simulink model "LUT_liver_pancreas_30"  (R2023b)
settings: Solver=FixedStepAuto  StartTime=0  StopTime=10.1  FixedStep=Timegap  RelTol=1e-3
model workspace (MAT data in the model file):
  T1_input = 1.34
(part 1 of 3)
settings Model: Creator=ppxmr2  LastModifiedBy=ppxmr2

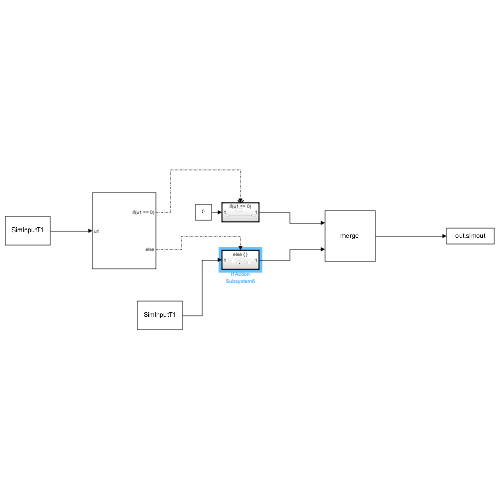
[thumbnail: Simulink's stored preview of the top-level diagram]
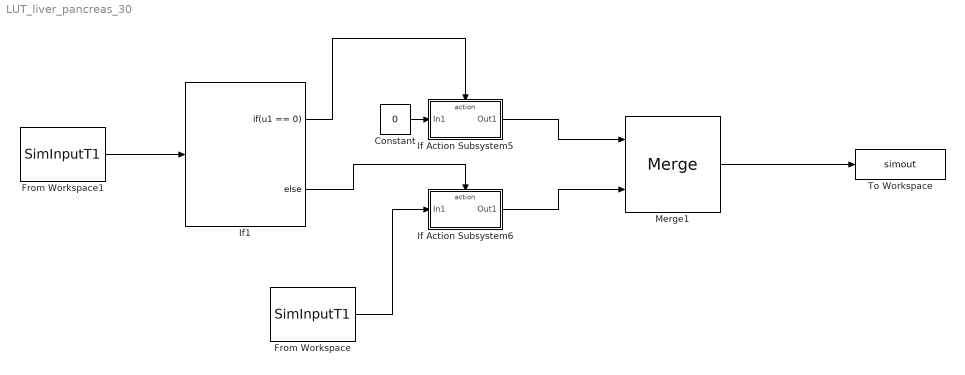
== system LUT_liver_pancreas_30 ==
  Constant : Constant  Value=0
  From Workspace : FromWorkspace  VariableName=SimInputT1  Interpolate=off  OutputAfterFinalValue=Setting to zero
  From Workspace1 : FromWorkspace  VariableName=SimInputT1  Interpolate=off  OutputAfterFinalValue=Setting to zero
  If Action Subsystem5 : Subsystem  TreatAsAtomicUnit=on
  If Action Subsystem6 : Subsystem  TreatAsAtomicUnit=on
  If1 : If  IfExpression=u1 == 0
  Merge1 : Merge
  To Workspace : ToWorkspace  VariableName=simout
  wires:
  From Workspace1/1 -> If1/1
  If1/1 -> If Action Subsystem5/Action
  If1/2 -> If Action Subsystem6/Action
  Constant/1 -> If Action Subsystem5/1(In1)
  If Action Subsystem5/1(Out1) -> Merge1/1
  If Action Subsystem6/1(Out1) -> Merge1/2
  Merge1/1 -> To Workspace/1
  From Workspace/1 -> If Action Subsystem6/1(In1)

== system LUT_liver_pancreas_30/If Action Subsystem5 ==
  In1 : Inport
  Action Port : ActionPort  ActionPortLabel=if(u1 == 0)
  Out1 : Outport
  wires:
  In1/1 -> Out1/1

== system LUT_liver_pancreas_30/If Action Subsystem6 ==
  In1 : Inport
  Action Port : ActionPort  ActionPortLabel=else
  From Workspace1 : FromWorkspace  VariableName=SimInputHR  Interpolate=off  OutputAfterFinalValue=Setting to zero
  If : If  IfExpression=u1 >= 1.495  ElseIfExpressions=u1 >= 0.995
  If Action Subsystem1 : Subsystem  TreatAsAtomicUnit=on
  If Action Subsystem2 : Subsystem  TreatAsAtomicUnit=on
  If Action Subsystem3 : Subsystem  TreatAsAtomicUnit=on
  Merge : Merge  Inputs=3
  Out1 : Outport
  wires:
  Merge/1 -> Out1/1
  From Workspace1/1 -> If/1
  If Action Subsystem1/1(Out1) -> Merge/2
  If Action Subsystem3/1(Out1) -> Merge/3
  In1/1 -> If Action Subsystem2/1(In1), If Action Subsystem1/1(In1), If Action Subsystem3/1(In1)
  If/1 -> If Action Subsystem2/Action
  If/2 -> If Action Subsystem1/Action
  If/3 -> If Action Subsystem3/Action
  If Action Subsystem2/1(Out1) -> Merge/1

== system LUT_liver_pancreas_30/If Action Subsystem6/If Action Subsystem1 ==
  In1 : Inport
  Action Port : ActionPort  ActionPortLabel=elseif(u1 >= 0.995)
  From Workspace2 : FromWorkspace  VariableName=SimInputHR  Interpolate=off  OutputAfterFinalValue=Setting to zero
  If Action Subsystem5 : Subsystem  TreatAsAtomicUnit=on
  If Action Subsystem6 : Subsystem  TreatAsAtomicUnit=on
  If Action Subsystem7 : Subsystem  TreatAsAtomicUnit=on
  If Action Subsystem8 : Subsystem  TreatAsAtomicUnit=on
  If Action Subsystem9 : Subsystem  TreatAsAtomicUnit=on
  If1 : If  IfExpression=u1 >= 1.395  ElseIfExpressions=u1 >= 1.295, u1 >= 1.195, u1 >= 1.095
  Merge1 : Merge  Inputs=5
  Out1 : Outport
  wires:
  In1/1 -> If Action Subsystem7/1(In2), If Action Subsystem8/1(In1), If Action Subsystem9/1(In1), If Action Subsystem5/1(In1), If Action Subsystem6/1(In1)
  From Workspace2/1 -> If1/1
  If Action Subsystem9/1(Out1) -> Merge1/1
  If Action Subsystem6/1(Out1) -> Merge1/5
  If Action Subsystem8/1(Out1) -> Merge1/2
  If Action Subsystem5/1(Out1) -> Merge1/4
  If1/4 -> If Action Subsystem5/Action
  If1/2 -> If Action Subsystem8/Action
  If1/3 -> If Action Subsystem7/Action
  If Action Subsystem7/1(Out2) -> Merge1/3
  If1/5 -> If Action Subsystem6/Action
  If1/1 -> If Action Subsystem9/Action
  Merge1/1 -> Out1/1

== system LUT_liver_pancreas_30/If Action Subsystem6/If Action Subsystem2 ==
  In1 : Inport
  Action Port : ActionPort  ActionPortLabel=if(u1 >= 1.495)
  From Workspace2 : FromWorkspace  VariableName=SimInputHR  Interpolate=off  OutputAfterFinalValue=Setting to zero
  If Action Subsystem5 : Subsystem  TreatAsAtomicUnit=on
  If Action Subsystem6 : Subsystem  TreatAsAtomicUnit=on
  If Action Subsystem7 : Subsystem  TreatAsAtomicUnit=on
  If Action Subsystem8 : Subsystem  TreatAsAtomicUnit=on
  If Action Subsystem9 : Subsystem  TreatAsAtomicUnit=on
  If1 : If  IfExpression=u1 >= 1.895  ElseIfExpressions=u1 >= 1.795, u1 >= 1.695, u1 >= 1.595
  Merge1 : Merge  Inputs=5
  Out1 : Outport
  wires:
  In1/1 -> If Action Subsystem9/1(In1), If Action Subsystem8/1(In1), If Action Subsystem7/1(In1), If Action Subsystem5/1(In1), If Action Subsystem6/1(In1)
  From Workspace2/1 -> If1/1
  If Action Subsystem9/1(Out1) -> Merge1/1
  If1/4 -> If Action Subsystem5/Action
  If1/2 -> If Action Subsystem8/Action
  If1/3 -> If Action Subsystem7/Action
  If1/5 -> If Action Subsystem6/Action
  If1/1 -> If Action Subsystem9/Action
  Merge1/1 -> Out1/1
  If Action Subsystem8/1(Out1) -> Merge1/2
  If Action Subsystem7/1(Out1) -> Merge1/3
  If Action Subsystem6/1(Out1) -> Merge1/5
  If Action Subsystem5/1(Out1) -> Merge1/4

== system LUT_liver_pancreas_30/If Action Subsystem6/If Action Subsystem3 ==
  In1 : Inport
  Action Port : ActionPort  ActionPortLabel=else
  From Workspace2 : FromWorkspace  VariableName=SimInputHR  Interpolate=off  OutputAfterFinalValue=Setting to zero
  If Action Subsystem5 : Subsystem  TreatAsAtomicUnit=on
  If Action Subsystem6 : Subsystem  TreatAsAtomicUnit=on
  If Action Subsystem7 : Subsystem  TreatAsAtomicUnit=on
  If Action Subsystem8 : Subsystem  TreatAsAtomicUnit=on
  If Action Subsystem9 : Subsystem  TreatAsAtomicUnit=on
  If1 : If  IfExpression=u1 >= 0.895  ElseIfExpressions=u1 >= 0.795, u1 >= 0.695, u1 >= 0595
  Merge1 : Merge  Inputs=5
  Out1 : Outport
  wires:
  In1/1 -> If Action Subsystem8/1(In1), If Action Subsystem9/1(In2), If Action Subsystem7/1(In1), If Action Subsystem5/1(In1), If Action Subsystem6/1(In1)
  From Workspace2/1 -> If1/1
  If Action Subsystem9/1(Out2) -> Merge1/1
  If Action Subsystem6/1(Out1) -> Merge1/5
  If Action Subsystem8/1(Out1) -> Merge1/2
  If Action Subsystem5/1(Out1) -> Merge1/4
  If1/4 -> If Action Subsystem5/Action
  If1/2 -> If Action Subsystem8/Action
  If1/3 -> If Action Subsystem7/Action
  If Action Subsystem7/1(Out1) -> Merge1/3
  If1/5 -> If Action Subsystem6/Action
  If1/1 -> If Action Subsystem9/Action
  Merge1/1 -> Out1/1

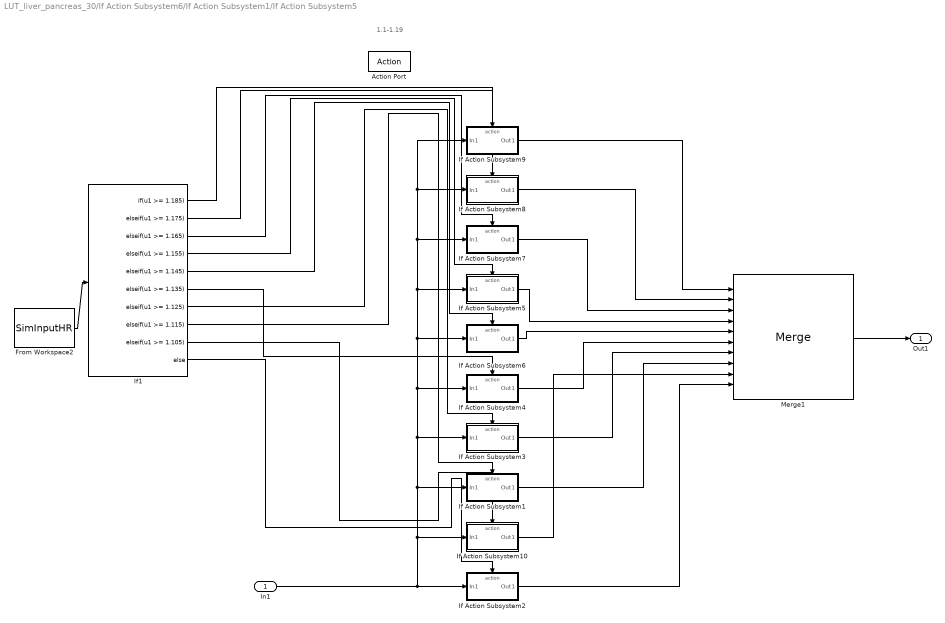
== system LUT_liver_pancreas_30/If Action Subsystem6/If Action Subsystem1/If Action Subsystem5 ==
  note: 1.1-1.19
  In1 : Inport
  Action Port : ActionPort  ActionPortLabel=elseif( u1 >= 1.095)
  From Workspace2 : FromWorkspace  VariableName=SimInputHR  Interpolate=off  OutputAfterFinalValue=Setting to zero
  If Action Subsystem1 : Subsystem  TreatAsAtomicUnit=on
  If Action Subsystem10 : Subsystem  TreatAsAtomicUnit=on
  If Action Subsystem2 : Subsystem  TreatAsAtomicUnit=on
  If Action Subsystem3 : Subsystem  TreatAsAtomicUnit=on
  If Action Subsystem4 : Subsystem  TreatAsAtomicUnit=on
  If Action Subsystem5 : Subsystem  TreatAsAtomicUnit=on
  If Action Subsystem6 : Subsystem  TreatAsAtomicUnit=on
  If Action Subsystem7 : Subsystem  TreatAsAtomicUnit=on
  If Action Subsystem8 : Subsystem  TreatAsAtomicUnit=on
  If Action Subsystem9 : Subsystem  TreatAsAtomicUnit=on
  If1 : If  IfExpression=u1 >= 1.185  ElseIfExpressions=u1 >= 1.175, u1 >= 1.165, u1 >= 1.155, u1 >= 1.145, u1 >= 1.135, u1 >= 1.125, u1 >= 1.115, u1 >= 1.105
  Merge1 : Merge  Inputs=10
  Out1 : Outport
  wires:
  If1/10 -> If Action Subsystem2/Action
  If Action Subsystem4/1(Out1) -> Merge1/6
  From Workspace2/1 -> If1/1
  If Action Subsystem6/1(Out1) -> Merge1/5
  Merge1/1 -> Out1/1
  If1/8 -> If Action Subsystem1/Action
  If Action Subsystem3/1(Out1) -> Merge1/7
  In1/1 -> If Action Subsystem1/1(In1), If Action Subsystem3/1(In1), If Action Subsystem7/1(In1), If Action Subsystem8/1(In1), If Action Subsystem9/1(In1), If Action Subsystem5/1(In1), If Action Subsystem6/1(In1), If Action Subsystem4/1(In1), If Action Subsystem10/1(In1), If Action Subsystem2/1(In1)
  If1/6 -> If Action Subsystem4/Action
  If Action Subsystem1/1(Out1) -> Merge1/8
  If1/4 -> If Action Subsystem5/Action
  If Action Subsystem8/1(Out1) -> Merge1/2
  If1/5 -> If Action Subsystem6/Action
  If Action Subsystem7/1(Out1) -> Merge1/3
  If1/3 -> If Action Subsystem7/Action
  If1/7 -> If Action Subsystem3/Action
  If Action Subsystem5/1(Out1) -> Merge1/4
  If Action Subsystem2/1(Out1) -> Merge1/10
  If1/2 -> If Action Subsystem8/Action
  If1/1 -> If Action Subsystem9/Action
  If Action Subsystem9/1(Out1) -> Merge1/1
  If1/9 -> If Action Subsystem10/Action
  If Action Subsystem10/1(Out1) -> Merge1/9

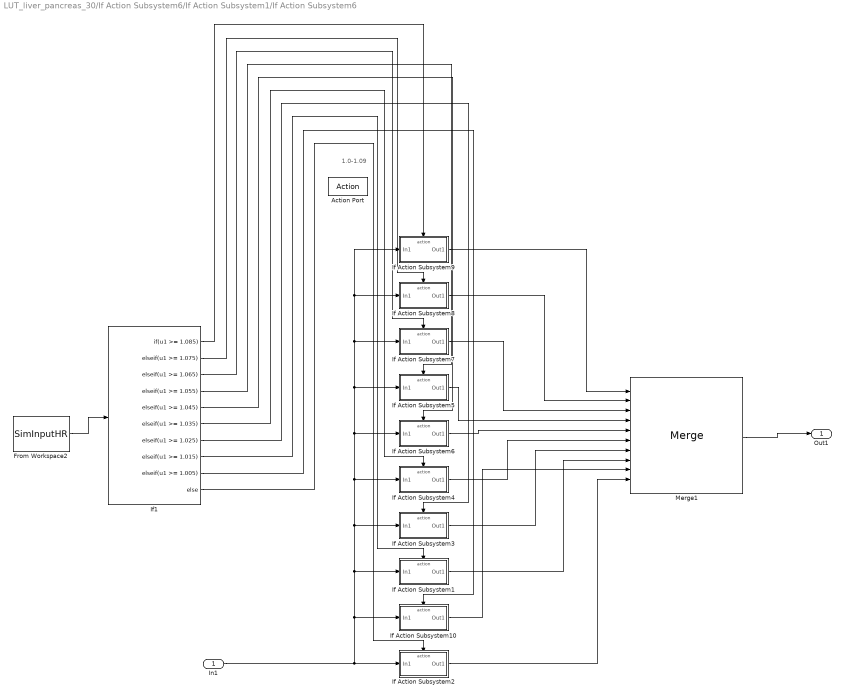
== system LUT_liver_pancreas_30/If Action Subsystem6/If Action Subsystem1/If Action Subsystem6 ==
  note: 1.0-1.09
  In1 : Inport
  Action Port : ActionPort  ActionPortLabel=else
  From Workspace2 : FromWorkspace  VariableName=SimInputHR  Interpolate=off  OutputAfterFinalValue=Setting to zero
  If Action Subsystem1 : Subsystem  TreatAsAtomicUnit=on
  If Action Subsystem10 : Subsystem  TreatAsAtomicUnit=on
  If Action Subsystem2 : Subsystem  TreatAsAtomicUnit=on
  If Action Subsystem3 : Subsystem  TreatAsAtomicUnit=on
  If Action Subsystem4 : Subsystem  TreatAsAtomicUnit=on
  If Action Subsystem5 : Subsystem  TreatAsAtomicUnit=on
  If Action Subsystem6 : Subsystem  TreatAsAtomicUnit=on
  If Action Subsystem7 : Subsystem  TreatAsAtomicUnit=on
  If Action Subsystem8 : Subsystem  TreatAsAtomicUnit=on
  If Action Subsystem9 : Subsystem  TreatAsAtomicUnit=on
  If1 : If  IfExpression=u1 >= 1.085  ElseIfExpressions=u1 >= 1.075, u1 >= 1.065, u1 >= 1.055, u1 >= 1.045, u1 >= 1.035, u1 >= 1.025, u1 >= 1.015, u1 >= 1.005
  Merge1 : Merge  Inputs=10
  Out1 : Outport
  wires:
  If1/10 -> If Action Subsystem2/Action
  If Action Subsystem4/1(Out1) -> Merge1/6
  From Workspace2/1 -> If1/1
  If Action Subsystem6/1(Out1) -> Merge1/5
  Merge1/1 -> Out1/1
  If1/8 -> If Action Subsystem1/Action
  If Action Subsystem3/1(Out1) -> Merge1/7
  In1/1 -> If Action Subsystem1/1(In1), If Action Subsystem3/1(In1), If Action Subsystem4/1(In1), If Action Subsystem7/1(In1), If Action Subsystem8/1(In1), If Action Subsystem9/1(In1), If Action Subsystem5/1(In1), If Action Subsystem6/1(In1), If Action Subsystem10/1(In1), If Action Subsystem2/1(In1)
  If1/6 -> If Action Subsystem4/Action
  If Action Subsystem1/1(Out1) -> Merge1/8
  If1/4 -> If Action Subsystem5/Action
  If Action Subsystem8/1(Out1) -> Merge1/2
  If1/5 -> If Action Subsystem6/Action
  If Action Subsystem7/1(Out1) -> Merge1/3
  If1/3 -> If Action Subsystem7/Action
  If1/7 -> If Action Subsystem3/Action
  If Action Subsystem5/1(Out1) -> Merge1/4
  If Action Subsystem2/1(Out1) -> Merge1/10
  If1/2 -> If Action Subsystem8/Action
  If1/1 -> If Action Subsystem9/Action
  If Action Subsystem9/1(Out1) -> Merge1/1
  If1/9 -> If Action Subsystem10/Action
  If Action Subsystem10/1(Out1) -> Merge1/9

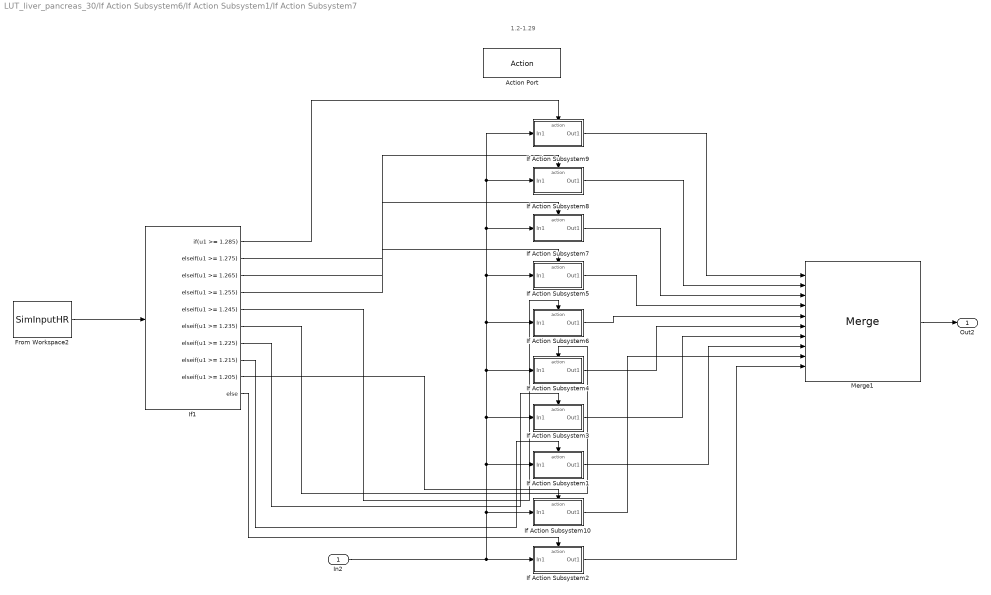
== system LUT_liver_pancreas_30/If Action Subsystem6/If Action Subsystem1/If Action Subsystem7 ==
  note: 1.2-1.29
  In2 : Inport
  Action Port : ActionPort  ActionPortLabel=elseif( u1 >= 1.195)
  From Workspace2 : FromWorkspace  VariableName=SimInputHR  Interpolate=off  OutputAfterFinalValue=Setting to zero
  If Action Subsystem1 : Subsystem  TreatAsAtomicUnit=on
  If Action Subsystem10 : Subsystem  TreatAsAtomicUnit=on
  If Action Subsystem2 : Subsystem  TreatAsAtomicUnit=on
  If Action Subsystem3 : Subsystem  TreatAsAtomicUnit=on
  If Action Subsystem4 : Subsystem  TreatAsAtomicUnit=on
  If Action Subsystem5 : Subsystem  TreatAsAtomicUnit=on
  If Action Subsystem6 : Subsystem  TreatAsAtomicUnit=on
  If Action Subsystem7 : Subsystem  TreatAsAtomicUnit=on
  If Action Subsystem8 : Subsystem  TreatAsAtomicUnit=on
  If Action Subsystem9 : Subsystem  TreatAsAtomicUnit=on
  If1 : If  IfExpression=u1 >= 1.285  ElseIfExpressions=u1 >= 1.275, u1 >= 1.265, u1 >= 1.255, u1 >= 1.245, u1 >= 1.235, u1 >= 1.225, u1 >= 1.215, u1 >= 1.205
  Merge1 : Merge  Inputs=10
  Out2 : Outport
  wires:
  If1/10 -> If Action Subsystem2/Action
  If Action Subsystem4/1(Out1) -> Merge1/6
  From Workspace2/1 -> If1/1
  If Action Subsystem6/1(Out1) -> Merge1/5
  Merge1/1 -> Out2/1
  If1/8 -> If Action Subsystem1/Action
  If Action Subsystem3/1(Out1) -> Merge1/7
  In2/1 -> If Action Subsystem1/1(In1), If Action Subsystem3/1(In1), If Action Subsystem4/1(In1), If Action Subsystem7/1(In1), If Action Subsystem8/1(In1), If Action Subsystem9/1(In1), If Action Subsystem5/1(In1), If Action Subsystem6/1(In1), If Action Subsystem10/1(In1), If Action Subsystem2/1(In1)
  If1/6 -> If Action Subsystem4/Action
  If Action Subsystem1/1(Out1) -> Merge1/8
  If1/4 -> If Action Subsystem5/Action
  If Action Subsystem8/1(Out1) -> Merge1/2
  If1/5 -> If Action Subsystem6/Action
  If Action Subsystem7/1(Out1) -> Merge1/3
  If1/3 -> If Action Subsystem7/Action
  If1/7 -> If Action Subsystem3/Action
  If Action Subsystem5/1(Out1) -> Merge1/4
  If Action Subsystem2/1(Out1) -> Merge1/10
  If1/2 -> If Action Subsystem8/Action
  If1/1 -> If Action Subsystem9/Action
  If Action Subsystem9/1(Out1) -> Merge1/1
  If Action Subsystem10/1(Out1) -> Merge1/9
  If1/9 -> If Action Subsystem10/Action

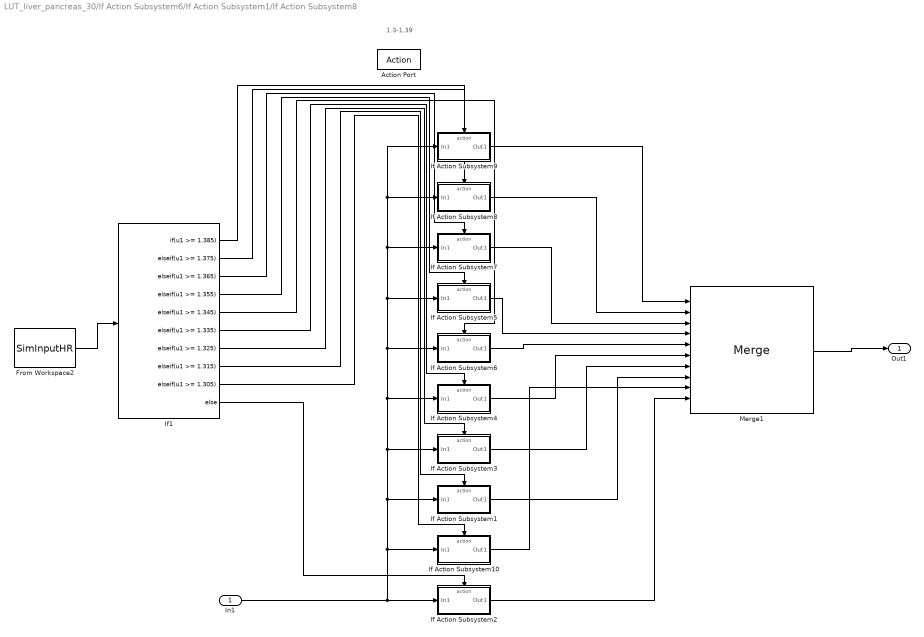
== system LUT_liver_pancreas_30/If Action Subsystem6/If Action Subsystem1/If Action Subsystem8 ==
  note: 1.3-1.39
  In1 : Inport
  Action Port : ActionPort  ActionPortLabel=elseif(u1 >= 1.295)
  From Workspace2 : FromWorkspace  VariableName=SimInputHR  Interpolate=off  OutputAfterFinalValue=Setting to zero
  If Action Subsystem1 : Subsystem  TreatAsAtomicUnit=on
  If Action Subsystem10 : Subsystem  TreatAsAtomicUnit=on
  If Action Subsystem2 : Subsystem  TreatAsAtomicUnit=on
  If Action Subsystem3 : Subsystem  TreatAsAtomicUnit=on
  If Action Subsystem4 : Subsystem  TreatAsAtomicUnit=on
  If Action Subsystem5 : Subsystem  TreatAsAtomicUnit=on
  If Action Subsystem6 : Subsystem  TreatAsAtomicUnit=on
  If Action Subsystem7 : Subsystem  TreatAsAtomicUnit=on
  If Action Subsystem8 : Subsystem  TreatAsAtomicUnit=on
  If Action Subsystem9 : Subsystem  TreatAsAtomicUnit=on
  If1 : If  IfExpression=u1 >= 1.385  ElseIfExpressions=u1 >= 1.375, u1 >= 1.365, u1 >= 1.355, u1 >= 1.345, u1 >= 1.335, u1 >= 1.325, u1 >= 1.315, u1 >= 1.305
  Merge1 : Merge  Inputs=10
  Out1 : Outport
  wires:
  If1/10 -> If Action Subsystem2/Action
  If Action Subsystem4/1(Out1) -> Merge1/6
  From Workspace2/1 -> If1/1
  If Action Subsystem6/1(Out1) -> Merge1/5
  Merge1/1 -> Out1/1
  If1/8 -> If Action Subsystem1/Action
  If Action Subsystem3/1(Out1) -> Merge1/7
  In1/1 -> If Action Subsystem1/1(In1), If Action Subsystem3/1(In1), If Action Subsystem4/1(In1), If Action Subsystem7/1(In1), If Action Subsystem8/1(In1), If Action Subsystem9/1(In1), If Action Subsystem5/1(In1), If Action Subsystem6/1(In1), If Action Subsystem10/1(In1), If Action Subsystem2/1(In1)
  If1/6 -> If Action Subsystem4/Action
  If Action Subsystem1/1(Out1) -> Merge1/8
  If1/4 -> If Action Subsystem5/Action
  If Action Subsystem8/1(Out1) -> Merge1/2
  If1/5 -> If Action Subsystem6/Action
  If Action Subsystem7/1(Out1) -> Merge1/3
  If1/3 -> If Action Subsystem7/Action
  If1/7 -> If Action Subsystem3/Action
  If Action Subsystem5/1(Out1) -> Merge1/4
  If Action Subsystem2/1(Out1) -> Merge1/10
  If1/2 -> If Action Subsystem8/Action
  If1/1 -> If Action Subsystem9/Action
  If Action Subsystem9/1(Out1) -> Merge1/1
  If1/9 -> If Action Subsystem10/Action
  If Action Subsystem10/1(Out1) -> Merge1/9

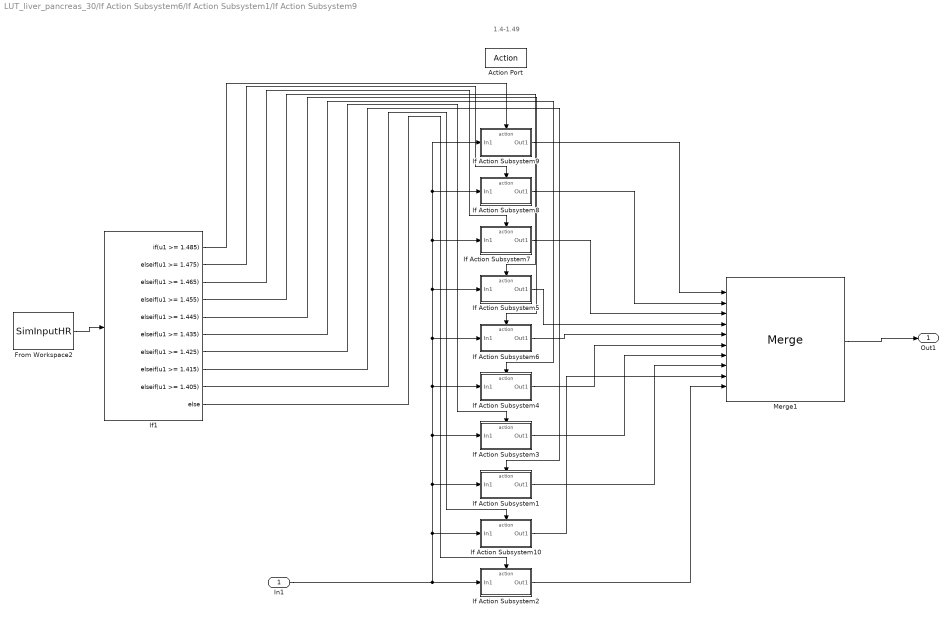
== system LUT_liver_pancreas_30/If Action Subsystem6/If Action Subsystem1/If Action Subsystem9 ==
  note: 1.4-1.49
  In1 : Inport
  Action Port : ActionPort  ActionPortLabel=if(u1 >= 1.395)
  From Workspace2 : FromWorkspace  VariableName=SimInputHR  Interpolate=off  OutputAfterFinalValue=Setting to zero
  If Action Subsystem1 : Subsystem  TreatAsAtomicUnit=on
  If Action Subsystem10 : Subsystem  TreatAsAtomicUnit=on
  If Action Subsystem2 : Subsystem  TreatAsAtomicUnit=on
  If Action Subsystem3 : Subsystem  TreatAsAtomicUnit=on
  If Action Subsystem4 : Subsystem  TreatAsAtomicUnit=on
  If Action Subsystem5 : Subsystem  TreatAsAtomicUnit=on
  If Action Subsystem6 : Subsystem  TreatAsAtomicUnit=on
  If Action Subsystem7 : Subsystem  TreatAsAtomicUnit=on
  If Action Subsystem8 : Subsystem  TreatAsAtomicUnit=on
  If Action Subsystem9 : Subsystem  TreatAsAtomicUnit=on
  If1 : If  IfExpression=u1 >= 1.485  ElseIfExpressions=u1 >= 1.475, u1 >= 1.465, u1 >= 1.455, u1 >= 1.445, u1 >= 1.435, u1 >= 1.425, u1 >= 1.415, u1 >= 1.405
  Merge1 : Merge  Inputs=10
  Out1 : Outport
  wires:
  If1/10 -> If Action Subsystem2/Action
  If Action Subsystem4/1(Out1) -> Merge1/6
  From Workspace2/1 -> If1/1
  If Action Subsystem6/1(Out1) -> Merge1/5
  Merge1/1 -> Out1/1
  If1/8 -> If Action Subsystem1/Action
  If Action Subsystem3/1(Out1) -> Merge1/7
  In1/1 -> If Action Subsystem10/1(In1), If Action Subsystem1/1(In1), If Action Subsystem3/1(In1), If Action Subsystem4/1(In1), If Action Subsystem7/1(In1), If Action Subsystem8/1(In1), If Action Subsystem9/1(In1), If Action Subsystem5/1(In1), If Action Subsystem6/1(In1), If Action Subsystem2/1(In1)
  If1/6 -> If Action Subsystem4/Action
  If Action Subsystem1/1(Out1) -> Merge1/8
  If1/4 -> If Action Subsystem5/Action
  If Action Subsystem8/1(Out1) -> Merge1/2
  If1/5 -> If Action Subsystem6/Action
  If Action Subsystem7/1(Out1) -> Merge1/3
  If1/3 -> If Action Subsystem7/Action
  If1/7 -> If Action Subsystem3/Action
  If Action Subsystem5/1(Out1) -> Merge1/4
  If Action Subsystem2/1(Out1) -> Merge1/10
  If1/2 -> If Action Subsystem8/Action
  If1/1 -> If Action Subsystem9/Action
  If Action Subsystem9/1(Out1) -> Merge1/1
  If1/9 -> If Action Subsystem10/Action
  If Action Subsystem10/1(Out1) -> Merge1/9

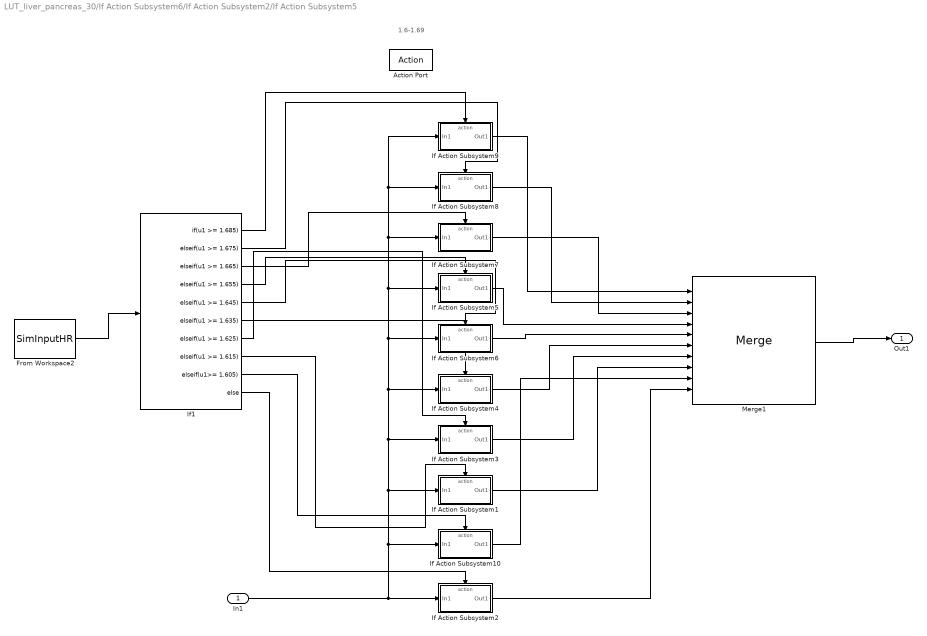
== system LUT_liver_pancreas_30/If Action Subsystem6/If Action Subsystem2/If Action Subsystem5 ==
  note: 1.6-1.69
  In1 : Inport
  Action Port : ActionPort  ActionPortLabel=elseif( u1 >= 1.595)
  From Workspace2 : FromWorkspace  VariableName=SimInputHR  Interpolate=off  OutputAfterFinalValue=Setting to zero
  If Action Subsystem1 : Subsystem  TreatAsAtomicUnit=on
  If Action Subsystem10 : Subsystem  TreatAsAtomicUnit=on
  If Action Subsystem2 : Subsystem  TreatAsAtomicUnit=on
  If Action Subsystem3 : Subsystem  TreatAsAtomicUnit=on
  If Action Subsystem4 : Subsystem  TreatAsAtomicUnit=on
  If Action Subsystem5 : Subsystem  TreatAsAtomicUnit=on
  If Action Subsystem6 : Subsystem  TreatAsAtomicUnit=on
  If Action Subsystem7 : Subsystem  TreatAsAtomicUnit=on
  If Action Subsystem8 : Subsystem  TreatAsAtomicUnit=on
  If Action Subsystem9 : Subsystem  TreatAsAtomicUnit=on
  If1 : If  IfExpression=u1 >= 1.685  ElseIfExpressions=u1 >= 1.675, u1 >= 1.665, u1 >= 1.655, u1 >= 1.645, u1 >= 1.635, u1 >= 1.625, u1 >= 1.615, u1>= 1.605
  Merge1 : Merge  Inputs=10
  Out1 : Outport
  wires:
  If1/2 -> If Action Subsystem8/Action
  If Action Subsystem5/1(Out1) -> Merge1/4
  If1/3 -> If Action Subsystem7/Action
  If Action Subsystem9/1(Out1) -> Merge1/1
  If1/7 -> If Action Subsystem3/Action
  If1/5 -> If Action Subsystem6/Action
  If1/1 -> If Action Subsystem9/Action
  If Action Subsystem4/1(Out1) -> Merge1/6
  If1/10 -> If Action Subsystem2/Action
  If Action Subsystem8/1(Out1) -> Merge1/2
  If1/4 -> If Action Subsystem5/Action
  In1/1 -> If Action Subsystem10/1(In1), If Action Subsystem1/1(In1), If Action Subsystem3/1(In1), If Action Subsystem4/1(In1), If Action Subsystem7/1(In1), If Action Subsystem8/1(In1), If Action Subsystem9/1(In1), If Action Subsystem5/1(In1), If Action Subsystem6/1(In1), If Action Subsystem2/1(In1)
  If Action Subsystem1/1(Out1) -> Merge1/8
  If Action Subsystem2/1(Out1) -> Merge1/10
  If1/8 -> If Action Subsystem1/Action
  If Action Subsystem3/1(Out1) -> Merge1/7
  If1/6 -> If Action Subsystem4/Action
  From Workspace2/1 -> If1/1
  Merge1/1 -> Out1/1
  If Action Subsystem6/1(Out1) -> Merge1/5
  If Action Subsystem7/1(Out1) -> Merge1/3
  If1/9 -> If Action Subsystem10/Action
  If Action Subsystem10/1(Out1) -> Merge1/9

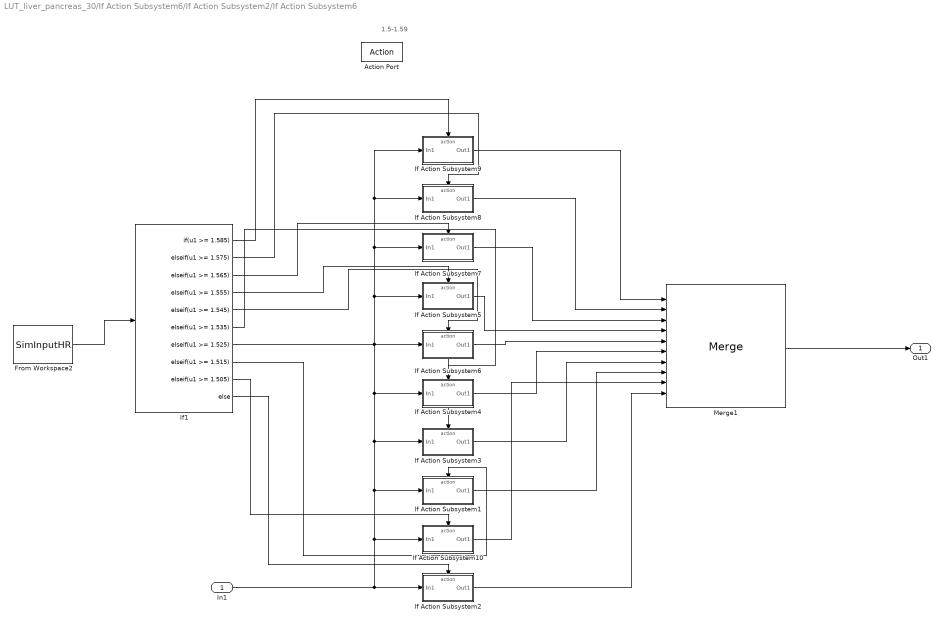
== system LUT_liver_pancreas_30/If Action Subsystem6/If Action Subsystem2/If Action Subsystem6 ==
  note: 1.5-1.59
  In1 : Inport
  Action Port : ActionPort  ActionPortLabel=else
  From Workspace2 : FromWorkspace  VariableName=SimInputHR  Interpolate=off  OutputAfterFinalValue=Setting to zero
  If Action Subsystem1 : Subsystem  TreatAsAtomicUnit=on
  If Action Subsystem10 : Subsystem  TreatAsAtomicUnit=on
  If Action Subsystem2 : Subsystem  TreatAsAtomicUnit=on
  If Action Subsystem3 : Subsystem  TreatAsAtomicUnit=on
  If Action Subsystem4 : Subsystem  TreatAsAtomicUnit=on
  If Action Subsystem5 : Subsystem  TreatAsAtomicUnit=on
  If Action Subsystem6 : Subsystem  TreatAsAtomicUnit=on
  If Action Subsystem7 : Subsystem  TreatAsAtomicUnit=on
  If Action Subsystem8 : Subsystem  TreatAsAtomicUnit=on
  If Action Subsystem9 : Subsystem  TreatAsAtomicUnit=on
  If1 : If  IfExpression=u1 >= 1.585  ElseIfExpressions=u1 >= 1.575, u1 >= 1.565, u1 >= 1.555, u1 >= 1.545, u1 >= 1.535, u1 >= 1.525, u1 >= 1.515, u1 >= 1.505
  Merge1 : Merge  Inputs=10
  Out1 : Outport
  wires:
  If1/2 -> If Action Subsystem8/Action
  If Action Subsystem5/1(Out1) -> Merge1/4
  If1/3 -> If Action Subsystem7/Action
  If Action Subsystem9/1(Out1) -> Merge1/1
  If1/7 -> If Action Subsystem3/Action
  If1/5 -> If Action Subsystem6/Action
  If1/1 -> If Action Subsystem9/Action
  If Action Subsystem4/1(Out1) -> Merge1/6
  If1/10 -> If Action Subsystem2/Action
  If Action Subsystem8/1(Out1) -> Merge1/2
  If1/4 -> If Action Subsystem5/Action
  In1/1 -> If Action Subsystem10/1(In1), If Action Subsystem1/1(In1), If Action Subsystem3/1(In1), If Action Subsystem4/1(In1), If Action Subsystem7/1(In1), If Action Subsystem8/1(In1), If Action Subsystem9/1(In1), If Action Subsystem5/1(In1), If Action Subsystem6/1(In1), If Action Subsystem2/1(In1)
  If Action Subsystem1/1(Out1) -> Merge1/8
  If Action Subsystem2/1(Out1) -> Merge1/10
  If1/8 -> If Action Subsystem1/Action
  If Action Subsystem3/1(Out1) -> Merge1/7
  If1/6 -> If Action Subsystem4/Action
  From Workspace2/1 -> If1/1
  Merge1/1 -> Out1/1
  If Action Subsystem6/1(Out1) -> Merge1/5
  If Action Subsystem7/1(Out1) -> Merge1/3
  If1/9 -> If Action Subsystem10/Action
  If Action Subsystem10/1(Out1) -> Merge1/9

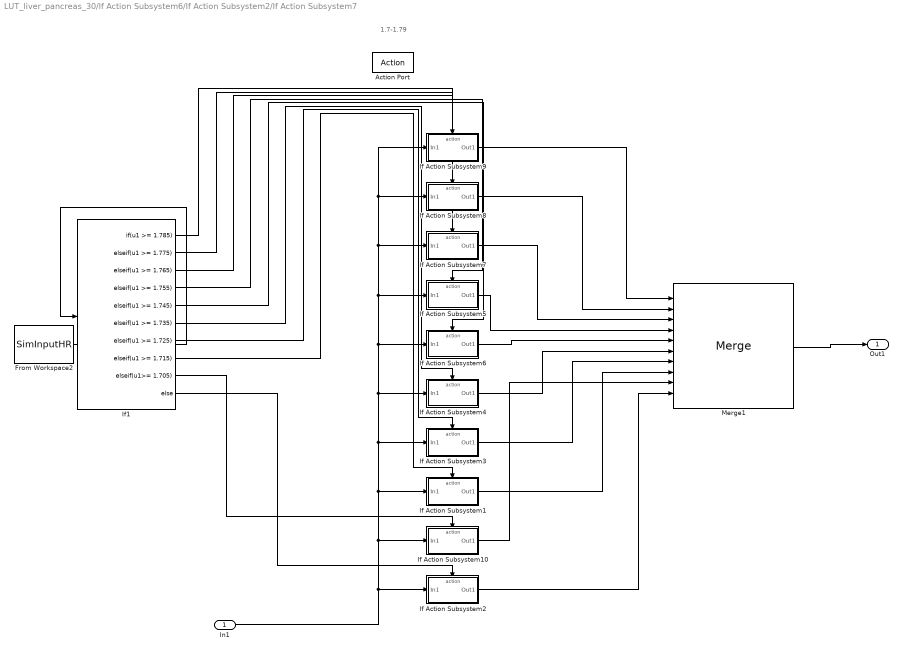
== system LUT_liver_pancreas_30/If Action Subsystem6/If Action Subsystem2/If Action Subsystem7 ==
  note: 1.7-1.79
  In1 : Inport
  Action Port : ActionPort  ActionPortLabel=elseif( u1 >= 1.695)
  From Workspace2 : FromWorkspace  VariableName=SimInputHR  Interpolate=off  OutputAfterFinalValue=Setting to zero
  If Action Subsystem1 : Subsystem  TreatAsAtomicUnit=on
  If Action Subsystem10 : Subsystem  TreatAsAtomicUnit=on
  If Action Subsystem2 : Subsystem  TreatAsAtomicUnit=on
  If Action Subsystem3 : Subsystem  TreatAsAtomicUnit=on
  If Action Subsystem4 : Subsystem  TreatAsAtomicUnit=on
  If Action Subsystem5 : Subsystem  TreatAsAtomicUnit=on
  If Action Subsystem6 : Subsystem  TreatAsAtomicUnit=on
  If Action Subsystem7 : Subsystem  TreatAsAtomicUnit=on
  If Action Subsystem8 : Subsystem  TreatAsAtomicUnit=on
  If Action Subsystem9 : Subsystem  TreatAsAtomicUnit=on
  If1 : If  IfExpression=u1 >= 1.785  ElseIfExpressions=u1 >= 1.775, u1 >= 1.765, u1 >= 1.755, u1 >= 1.745, u1 >= 1.735, u1 >= 1.725, u1 >= 1.715, u1>= 1.705
  Merge1 : Merge  Inputs=10
  Out1 : Outport
  wires:
  If1/2 -> If Action Subsystem8/Action
  If Action Subsystem5/1(Out1) -> Merge1/4
  If1/3 -> If Action Subsystem7/Action
  If Action Subsystem9/1(Out1) -> Merge1/1
  If1/7 -> If Action Subsystem3/Action
  If1/5 -> If Action Subsystem6/Action
  If1/1 -> If Action Subsystem9/Action
  If Action Subsystem4/1(Out1) -> Merge1/6
  If1/10 -> If Action Subsystem2/Action
  If Action Subsystem8/1(Out1) -> Merge1/2
  If1/4 -> If Action Subsystem5/Action
  In1/1 -> If Action Subsystem10/1(In1), If Action Subsystem1/1(In1), If Action Subsystem3/1(In1), If Action Subsystem4/1(In1), If Action Subsystem7/1(In1), If Action Subsystem8/1(In1), If Action Subsystem9/1(In1), If Action Subsystem5/1(In1), If Action Subsystem6/1(In1), If Action Subsystem2/1(In1)
  If Action Subsystem1/1(Out1) -> Merge1/8
  If Action Subsystem2/1(Out1) -> Merge1/10
  If1/8 -> If Action Subsystem1/Action
  If Action Subsystem3/1(Out1) -> Merge1/7
  If1/6 -> If Action Subsystem4/Action
  From Workspace2/1 -> If1/1
  Merge1/1 -> Out1/1
  If Action Subsystem6/1(Out1) -> Merge1/5
  If Action Subsystem7/1(Out1) -> Merge1/3
  If Action Subsystem10/1(Out1) -> Merge1/9
  If1/9 -> If Action Subsystem10/Action

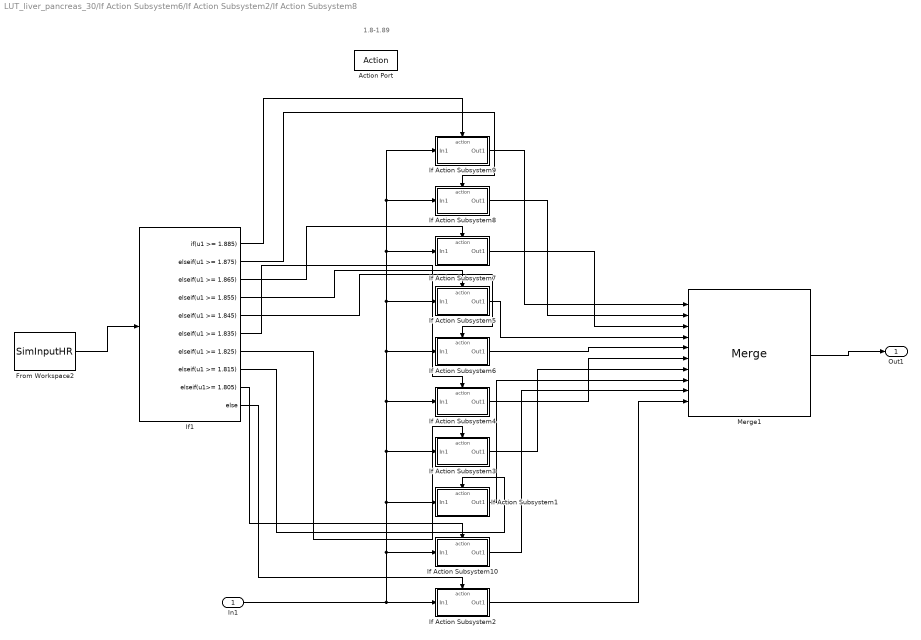
== system LUT_liver_pancreas_30/If Action Subsystem6/If Action Subsystem2/If Action Subsystem8 ==
  note: 1.8-1.89
  In1 : Inport
  Action Port : ActionPort  ActionPortLabel=elseif(u1 >= 1.795)
  From Workspace2 : FromWorkspace  VariableName=SimInputHR  Interpolate=off  OutputAfterFinalValue=Setting to zero
  If Action Subsystem1 : Subsystem  TreatAsAtomicUnit=on
  If Action Subsystem10 : Subsystem  TreatAsAtomicUnit=on
  If Action Subsystem2 : Subsystem  TreatAsAtomicUnit=on
  If Action Subsystem3 : Subsystem  TreatAsAtomicUnit=on
  If Action Subsystem4 : Subsystem  TreatAsAtomicUnit=on
  If Action Subsystem5 : Subsystem  TreatAsAtomicUnit=on
  If Action Subsystem6 : Subsystem  TreatAsAtomicUnit=on
  If Action Subsystem7 : Subsystem  TreatAsAtomicUnit=on
  If Action Subsystem8 : Subsystem  TreatAsAtomicUnit=on
  If Action Subsystem9 : Subsystem  TreatAsAtomicUnit=on
  If1 : If  IfExpression=u1 >= 1.885  ElseIfExpressions=u1 >= 1.875, u1 >= 1.865, u1 >= 1.855, u1 >= 1.845, u1 >= 1.835, u1 >= 1.825, u1 >= 1.815, u1>= 1.805
  Merge1 : Merge  Inputs=10
  Out1 : Outport
  wires:
  If1/2 -> If Action Subsystem8/Action
  If Action Subsystem5/1(Out1) -> Merge1/4
  If1/3 -> If Action Subsystem7/Action
  If Action Subsystem9/1(Out1) -> Merge1/1
  If1/7 -> If Action Subsystem3/Action
  If1/5 -> If Action Subsystem6/Action
  If1/1 -> If Action Subsystem9/Action
  If Action Subsystem4/1(Out1) -> Merge1/6
  If1/10 -> If Action Subsystem2/Action
  If Action Subsystem8/1(Out1) -> Merge1/2
  If1/4 -> If Action Subsystem5/Action
  In1/1 -> If Action Subsystem10/1(In1), If Action Subsystem1/1(In1), If Action Subsystem3/1(In1), If Action Subsystem4/1(In1), If Action Subsystem7/1(In1), If Action Subsystem8/1(In1), If Action Subsystem9/1(In1), If Action Subsystem5/1(In1), If Action Subsystem6/1(In1), If Action Subsystem2/1(In1)
  If Action Subsystem1/1(Out1) -> Merge1/8
  If Action Subsystem2/1(Out1) -> Merge1/10
  If1/8 -> If Action Subsystem1/Action
  If Action Subsystem3/1(Out1) -> Merge1/7
  If1/6 -> If Action Subsystem4/Action
  From Workspace2/1 -> If1/1
  Merge1/1 -> Out1/1
  If Action Subsystem6/1(Out1) -> Merge1/5
  If Action Subsystem7/1(Out1) -> Merge1/3
  If1/9 -> If Action Subsystem10/Action
  If Action Subsystem10/1(Out1) -> Merge1/9

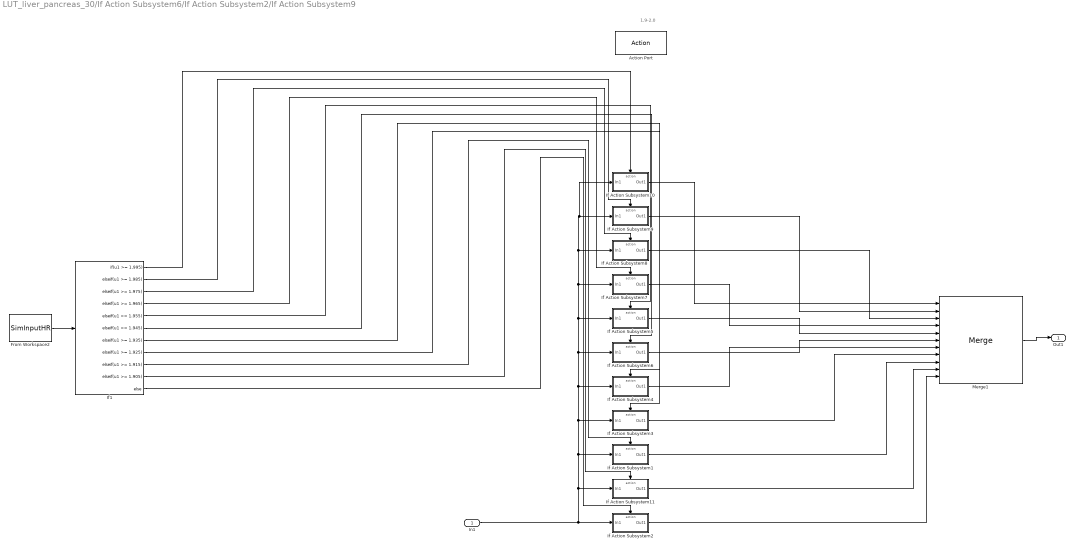
== system LUT_liver_pancreas_30/If Action Subsystem6/If Action Subsystem2/If Action Subsystem9 ==
  note: 1.9-2.0
  In1 : Inport
  Action Port : ActionPort  ActionPortLabel=if(u1 >= 1.895)
  From Workspace2 : FromWorkspace  VariableName=SimInputHR  Interpolate=off  OutputAfterFinalValue=Setting to zero
  If Action Subsystem1 : Subsystem  TreatAsAtomicUnit=on
  If Action Subsystem10 : Subsystem  TreatAsAtomicUnit=on
  If Action Subsystem11 : Subsystem  TreatAsAtomicUnit=on
  If Action Subsystem2 : Subsystem  TreatAsAtomicUnit=on
  If Action Subsystem3 : Subsystem  TreatAsAtomicUnit=on
  If Action Subsystem4 : Subsystem  TreatAsAtomicUnit=on
  If Action Subsystem5 : Subsystem  TreatAsAtomicUnit=on
  If Action Subsystem6 : Subsystem  TreatAsAtomicUnit=on
  If Action Subsystem7 : Subsystem  TreatAsAtomicUnit=on
  If Action Subsystem8 : Subsystem  TreatAsAtomicUnit=on
  If Action Subsystem9 : Subsystem  TreatAsAtomicUnit=on
  If1 : If  IfExpression=u1 >= 1.995  ElseIfExpressions=u1 >= 1.985, u1 >= 1.975, u1 >= 1.965, u1 >= 1.955, u1 >= 1.945, u1 >= 1.935, u1 >= 1.925, u1 >= 1.915, u1 >= 1.905
  Merge1 : Merge  Inputs=11
  Out1 : Outport
  wires:
  Merge1/1 -> Out1/1
  From Workspace2/1 -> If1/1
  If1/2 -> If Action Subsystem9/Action
  If1/3 -> If Action Subsystem8/Action
  If1/4 -> If Action Subsystem7/Action
  If1/5 -> If Action Subsystem5/Action
  If1/6 -> If Action Subsystem6/Action
  If1/7 -> If Action Subsystem4/Action
  If1/8 -> If Action Subsystem3/Action
  If1/9 -> If Action Subsystem1/Action
  If1/11 -> If Action Subsystem2/Action
  If Action Subsystem9/1(Out1) -> Merge1/2
  If Action Subsystem8/1(Out1) -> Merge1/3
  If Action Subsystem7/1(Out1) -> Merge1/4
  If Action Subsystem5/1(Out1) -> Merge1/5
  If Action Subsystem6/1(Out1) -> Merge1/6
  If Action Subsystem4/1(Out1) -> Merge1/7
  If Action Subsystem3/1(Out1) -> Merge1/8
  If Action Subsystem2/1(Out1) -> Merge1/11
  If Action Subsystem1/1(Out1) -> Merge1/9
  In1/1 -> If Action Subsystem1/1(In1), If Action Subsystem3/1(In1), If Action Subsystem4/1(In1), If Action Subsystem7/1(In1), If Action Subsystem8/1(In1), If Action Subsystem10/1(In1), If Action Subsystem9/1(In1), If Action Subsystem5/1(In1), If Action Subsystem6/1(In1), If Action Subsystem11/1(In1), If Action Subsystem2/1(In1)
  If1/1 -> If Action Subsystem10/Action
  If Action Subsystem10/1(Out1) -> Merge1/1
  If1/10 -> If Action Subsystem11/Action
  If Action Subsystem11/1(Out1) -> Merge1/10

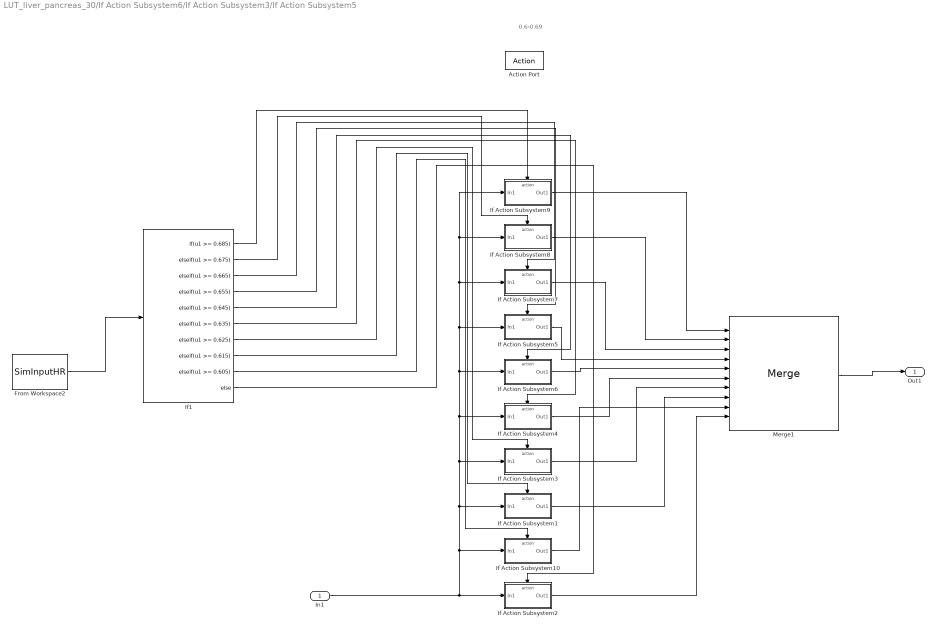
== system LUT_liver_pancreas_30/If Action Subsystem6/If Action Subsystem3/If Action Subsystem5 ==
  note: 0.6-0.69
  In1 : Inport
  Action Port : ActionPort  ActionPortLabel=elseif( u1 >= 0595)
  From Workspace2 : FromWorkspace  VariableName=SimInputHR  Interpolate=off  OutputAfterFinalValue=Setting to zero
  If Action Subsystem1 : Subsystem  TreatAsAtomicUnit=on
  If Action Subsystem10 : Subsystem  TreatAsAtomicUnit=on
  If Action Subsystem2 : Subsystem  TreatAsAtomicUnit=on
  If Action Subsystem3 : Subsystem  TreatAsAtomicUnit=on
  If Action Subsystem4 : Subsystem  TreatAsAtomicUnit=on
  If Action Subsystem5 : Subsystem  TreatAsAtomicUnit=on
  If Action Subsystem6 : Subsystem  TreatAsAtomicUnit=on
  If Action Subsystem7 : Subsystem  TreatAsAtomicUnit=on
  If Action Subsystem8 : Subsystem  TreatAsAtomicUnit=on
  If Action Subsystem9 : Subsystem  TreatAsAtomicUnit=on
  If1 : If  IfExpression=u1 >= 0.685  ElseIfExpressions=u1 >= 0.675, u1 >= 0.665, u1 >= 0.655, u1 >= 0.645, u1 >= 0.635, u1 >= 0.625, u1 >= 0.615, u1 >= 0.605
  Merge1 : Merge  Inputs=10
  Out1 : Outport
  wires:
  If1/10 -> If Action Subsystem2/Action
  If Action Subsystem4/1(Out1) -> Merge1/6
  From Workspace2/1 -> If1/1
  If Action Subsystem6/1(Out1) -> Merge1/5
  Merge1/1 -> Out1/1
  If1/8 -> If Action Subsystem1/Action
  If Action Subsystem3/1(Out1) -> Merge1/7
  In1/1 -> If Action Subsystem1/1(In1), If Action Subsystem3/1(In1), If Action Subsystem4/1(In1), If Action Subsystem7/1(In1), If Action Subsystem8/1(In1), If Action Subsystem9/1(In1), If Action Subsystem5/1(In1), If Action Subsystem6/1(In1), If Action Subsystem10/1(In1), If Action Subsystem2/1(In1)
  If1/6 -> If Action Subsystem4/Action
  If Action Subsystem1/1(Out1) -> Merge1/8
  If1/4 -> If Action Subsystem5/Action
  If Action Subsystem8/1(Out1) -> Merge1/2
  If1/5 -> If Action Subsystem6/Action
  If Action Subsystem7/1(Out1) -> Merge1/3
  If1/3 -> If Action Subsystem7/Action
  If1/7 -> If Action Subsystem3/Action
  If Action Subsystem5/1(Out1) -> Merge1/4
  If Action Subsystem2/1(Out1) -> Merge1/10
  If1/2 -> If Action Subsystem8/Action
  If1/1 -> If Action Subsystem9/Action
  If Action Subsystem9/1(Out1) -> Merge1/1
  If Action Subsystem10/1(Out1) -> Merge1/9
  If1/9 -> If Action Subsystem10/Action

== system LUT_liver_pancreas_30/If Action Subsystem6/If Action Subsystem3/If Action Subsystem6 ==
  note: 0.5-0.59
  In1 : Inport
  Action Port : ActionPort  ActionPortLabel=else
  From Workspace2 : FromWorkspace  VariableName=SimInputHR  Interpolate=off  OutputAfterFinalValue=Setting to zero
  If Action Subsystem1 : Subsystem  TreatAsAtomicUnit=on
  If Action Subsystem10 : Subsystem  TreatAsAtomicUnit=on
  If Action Subsystem2 : Subsystem  TreatAsAtomicUnit=on
  If Action Subsystem3 : Subsystem  TreatAsAtomicUnit=on
  If Action Subsystem4 : Subsystem  TreatAsAtomicUnit=on
  If Action Subsystem5 : Subsystem  TreatAsAtomicUnit=on
  If Action Subsystem6 : Subsystem  TreatAsAtomicUnit=on
  If Action Subsystem7 : Subsystem  TreatAsAtomicUnit=on
  If Action Subsystem8 : Subsystem  TreatAsAtomicUnit=on
  If Action Subsystem9 : Subsystem  TreatAsAtomicUnit=on
  If1 : If  IfExpression=u1 >= 0.585  ElseIfExpressions=u1 >= 0.575, u1 >= 0.565, u1 >= 0.555, u1 >= 0.545, u1 >= 0.535, u1 >= 0.525, u1 >= 0.515, u1 >= 0.505
  Merge1 : Merge  Inputs=10
  Out1 : Outport
  wires:
  If1/10 -> If Action Subsystem2/Action
  If Action Subsystem4/1(Out1) -> Merge1/6
  From Workspace2/1 -> If1/1
  If Action Subsystem6/1(Out1) -> Merge1/5
  Merge1/1 -> Out1/1
  If1/8 -> If Action Subsystem1/Action
  If Action Subsystem3/1(Out1) -> Merge1/7
  In1/1 -> If Action Subsystem1/1(In1), If Action Subsystem3/1(In1), If Action Subsystem4/1(In1), If Action Subsystem7/1(In1), If Action Subsystem8/1(In1), If Action Subsystem9/1(In1), If Action Subsystem5/1(In1), If Action Subsystem6/1(In1), If Action Subsystem10/1(In1), If Action Subsystem2/1(In1)
  If1/6 -> If Action Subsystem4/Action
  If Action Subsystem1/1(Out1) -> Merge1/8
  If1/4 -> If Action Subsystem5/Action
  If Action Subsystem8/1(Out1) -> Merge1/2
  If1/5 -> If Action Subsystem6/Action
  If Action Subsystem7/1(Out1) -> Merge1/3
  If1/3 -> If Action Subsystem7/Action
  If1/7 -> If Action Subsystem3/Action
  If Action Subsystem5/1(Out1) -> Merge1/4
  If Action Subsystem2/1(Out1) -> Merge1/10
  If1/2 -> If Action Subsystem8/Action
  If1/1 -> If Action Subsystem9/Action
  If Action Subsystem9/1(Out1) -> Merge1/1
  If Action Subsystem10/1(Out1) -> Merge1/9
  If1/9 -> If Action Subsystem10/Action

== system LUT_liver_pancreas_30/If Action Subsystem6/If Action Subsystem3/If Action Subsystem7 ==
  note: 0.7-0.79
  In1 : Inport
  Action Port : ActionPort  ActionPortLabel=elseif( u1 >= 0.695)
  From Workspace2 : FromWorkspace  VariableName=SimInputHR  Interpolate=off  OutputAfterFinalValue=Setting to zero
  If Action Subsystem1 : Subsystem  TreatAsAtomicUnit=on
  If Action Subsystem10 : Subsystem  TreatAsAtomicUnit=on
  If Action Subsystem2 : Subsystem  TreatAsAtomicUnit=on
  If Action Subsystem3 : Subsystem  TreatAsAtomicUnit=on
  If Action Subsystem4 : Subsystem  TreatAsAtomicUnit=on
  If Action Subsystem5 : Subsystem  TreatAsAtomicUnit=on
  If Action Subsystem6 : Subsystem  TreatAsAtomicUnit=on
  If Action Subsystem7 : Subsystem  TreatAsAtomicUnit=on
  If Action Subsystem8 : Subsystem  TreatAsAtomicUnit=on
  If Action Subsystem9 : Subsystem  TreatAsAtomicUnit=on
  If1 : If  IfExpression=u1 >= 0.785  ElseIfExpressions=u1 >= 0.775, u1 >= 0.765, u1 >= 0.755, u1 >= 0.745, u1 >= 0.735, u1 >= 0.725, u1 >= 0.715, u1 >= 0.705
  Merge1 : Merge  Inputs=10
  Out1 : Outport
  wires:
  If1/10 -> If Action Subsystem2/Action
  If Action Subsystem4/1(Out1) -> Merge1/6
  From Workspace2/1 -> If1/1
  If Action Subsystem6/1(Out1) -> Merge1/5
  Merge1/1 -> Out1/1
  If1/8 -> If Action Subsystem1/Action
  If Action Subsystem3/1(Out1) -> Merge1/7
  In1/1 -> If Action Subsystem1/1(In1), If Action Subsystem3/1(In1), If Action Subsystem4/1(In1), If Action Subsystem7/1(In1), If Action Subsystem8/1(In1), If Action Subsystem9/1(In1), If Action Subsystem5/1(In1), If Action Subsystem6/1(In1), If Action Subsystem10/1(In1), If Action Subsystem2/1(In1)
  If1/6 -> If Action Subsystem4/Action
  If Action Subsystem1/1(Out1) -> Merge1/8
  If1/4 -> If Action Subsystem5/Action
  If Action Subsystem8/1(Out1) -> Merge1/2
  If1/5 -> If Action Subsystem6/Action
  If Action Subsystem7/1(Out1) -> Merge1/3
  If1/3 -> If Action Subsystem7/Action
  If1/7 -> If Action Subsystem3/Action
  If Action Subsystem5/1(Out1) -> Merge1/4
  If Action Subsystem2/1(Out1) -> Merge1/10
  If1/2 -> If Action Subsystem8/Action
  If1/1 -> If Action Subsystem9/Action
  If Action Subsystem9/1(Out1) -> Merge1/1
  If1/9 -> If Action Subsystem10/Action
  If Action Subsystem10/1(Out1) -> Merge1/9

== system LUT_liver_pancreas_30/If Action Subsystem6/If Action Subsystem3/If Action Subsystem8 ==
  note: 0.8-0.89
  In1 : Inport
  Action Port : ActionPort  ActionPortLabel=elseif(u1 >= 0.795)
  From Workspace2 : FromWorkspace  VariableName=SimInputHR  Interpolate=off  OutputAfterFinalValue=Setting to zero
  If Action Subsystem1 : Subsystem  TreatAsAtomicUnit=on
  If Action Subsystem10 : Subsystem  TreatAsAtomicUnit=on
  If Action Subsystem2 : Subsystem  TreatAsAtomicUnit=on
  If Action Subsystem3 : Subsystem  TreatAsAtomicUnit=on
  If Action Subsystem4 : Subsystem  TreatAsAtomicUnit=on
  If Action Subsystem5 : Subsystem  TreatAsAtomicUnit=on
  If Action Subsystem6 : Subsystem  TreatAsAtomicUnit=on
  If Action Subsystem7 : Subsystem  TreatAsAtomicUnit=on
  If Action Subsystem8 : Subsystem  TreatAsAtomicUnit=on
  If Action Subsystem9 : Subsystem  TreatAsAtomicUnit=on
  If1 : If  IfExpression=u1 >= 0.885  ElseIfExpressions=u1 >= 0.875, u1 >= 0.865, u1 >= 0.855, u1 >= 0.845, u1 >= 0.835, u1 >= 0.825, u1 >= 0.815, u1 >= 0.805
  Merge1 : Merge  Inputs=10
  Out1 : Outport
  wires:
  If1/10 -> If Action Subsystem2/Action
  If Action Subsystem4/1(Out1) -> Merge1/6
  From Workspace2/1 -> If1/1
  If Action Subsystem6/1(Out1) -> Merge1/5
  Merge1/1 -> Out1/1
  If1/8 -> If Action Subsystem1/Action
  If Action Subsystem3/1(Out1) -> Merge1/7
  In1/1 -> If Action Subsystem1/1(In1), If Action Subsystem3/1(In1), If Action Subsystem4/1(In1), If Action Subsystem7/1(In1), If Action Subsystem8/1(In1), If Action Subsystem9/1(In1), If Action Subsystem5/1(In1), If Action Subsystem6/1(In1), If Action Subsystem10/1(In1), If Action Subsystem2/1(In1)
  If1/6 -> If Action Subsystem4/Action
  If Action Subsystem1/1(Out1) -> Merge1/8
  If1/4 -> If Action Subsystem5/Action
  If Action Subsystem8/1(Out1) -> Merge1/2
  If1/5 -> If Action Subsystem6/Action
  If Action Subsystem7/1(Out1) -> Merge1/3
  If1/3 -> If Action Subsystem7/Action
  If1/7 -> If Action Subsystem3/Action
  If Action Subsystem5/1(Out1) -> Merge1/4
  If Action Subsystem2/1(Out1) -> Merge1/10
  If1/2 -> If Action Subsystem8/Action
  If1/1 -> If Action Subsystem9/Action
  If Action Subsystem9/1(Out1) -> Merge1/1
  If1/9 -> If Action Subsystem10/Action
  If Action Subsystem10/1(Out1) -> Merge1/9

== system LUT_liver_pancreas_30/If Action Subsystem6/If Action Subsystem3/If Action Subsystem9 ==
  note: 0.9-0.99
  In2 : Inport
  Action Port : ActionPort  ActionPortLabel=if(u1 >= 0.895)
  From Workspace2 : FromWorkspace  VariableName=SimInputHR  Interpolate=off  OutputAfterFinalValue=Setting to zero
  If Action Subsystem1 : Subsystem  TreatAsAtomicUnit=on
  If Action Subsystem10 : Subsystem  TreatAsAtomicUnit=on
  If Action Subsystem2 : Subsystem  TreatAsAtomicUnit=on
  If Action Subsystem3 : Subsystem  TreatAsAtomicUnit=on
  If Action Subsystem4 : Subsystem  TreatAsAtomicUnit=on
  If Action Subsystem5 : Subsystem  TreatAsAtomicUnit=on
  If Action Subsystem6 : Subsystem  TreatAsAtomicUnit=on
  If Action Subsystem7 : Subsystem  TreatAsAtomicUnit=on
  If Action Subsystem8 : Subsystem  TreatAsAtomicUnit=on
  If Action Subsystem9 : Subsystem  TreatAsAtomicUnit=on
  If1 : If  IfExpression=u1 >= 0.985  ElseIfExpressions=u1 >= 0.975, u1 >= 0.965, u1 >= 0.955, u1 >= 0.945, u1 >= 0.935, u1 >= 0.925, u1 >= 0.915, u1 >= 0.905
  Merge1 : Merge  Inputs=10
  Out2 : Outport
  wires:
  If1/10 -> If Action Subsystem2/Action
  If Action Subsystem4/1(Out1) -> Merge1/6
  From Workspace2/1 -> If1/1
  If Action Subsystem6/1(Out1) -> Merge1/5
  Merge1/1 -> Out2/1
  If1/8 -> If Action Subsystem1/Action
  If Action Subsystem3/1(Out1) -> Merge1/7
  In2/1 -> If Action Subsystem10/1(In1), If Action Subsystem1/1(In1), If Action Subsystem3/1(In1), If Action Subsystem4/1(In1), If Action Subsystem7/1(In1), If Action Subsystem8/1(In1), If Action Subsystem9/1(In1), If Action Subsystem5/1(In1), If Action Subsystem6/1(In1), If Action Subsystem2/1(In1)
  If1/6 -> If Action Subsystem4/Action
  If Action Subsystem1/1(Out1) -> Merge1/8
  If1/4 -> If Action Subsystem5/Action
  If Action Subsystem8/1(Out1) -> Merge1/2
  If1/5 -> If Action Subsystem6/Action
  If Action Subsystem7/1(Out1) -> Merge1/3
  If1/3 -> If Action Subsystem7/Action
  If1/7 -> If Action Subsystem3/Action
  If Action Subsystem5/1(Out1) -> Merge1/4
  If Action Subsystem2/1(Out1) -> Merge1/10
  If1/2 -> If Action Subsystem8/Action
  If1/1 -> If Action Subsystem9/Action
  If Action Subsystem9/1(Out1) -> Merge1/1
  If1/9 -> If Action Subsystem10/Action
  If Action Subsystem10/1(Out1) -> Merge1/9

== system LUT_liver_pancreas_30/If Action Subsystem6/If Action Subsystem1/If Action Subsystem5/If Action Subsystem1 ==
  In1 : Inport
  Action Port : ActionPort  ActionPortLabel=elseif( u1 >= 1.115)
  LUT 1.12RR : Lookup_n-D  NumberOfTableDimensions=1  BreakpointsForDimension1=[463.9927;512.1024;609.3708;706.9796;804.4876;901.8858;999.198;1096.446;1193.646;1290.809;1387.943;1485.053;1582.145;1679.221;1776.281;1873.327;1970.357]  Table=[400;500;600;700;800;900;1000;1100;1200;1300;1400;1500;1600;1700;1800;1900;2000]  InternalRulePriority=Speed  RndMeth=Simplest
  Out1 : Outport
  wires:
  In1/1 -> LUT 1.12RR/1
  LUT 1.12RR/1 -> Out1/1

== system LUT_liver_pancreas_30/If Action Subsystem6/If Action Subsystem1/If Action Subsystem5/If Action Subsystem10 ==
  In1 : Inport
  Action Port : ActionPort  ActionPortLabel=elseif( u1 >= 1.105)
  LUT 1.11RR : Lookup_n-D  NumberOfTableDimensions=1  BreakpointsForDimension1=[464.1685;512.2902;609.641;707.3412;804.9463;902.4451;999.8606;1097.214;1194.52;1291.789;1389.031;1486.25;1583.451;1680.635;1777.804;1874.959;1972.096]  Table=[400;500;600;700;800;900;1000;1100;1200;1300;1400;1500;1600;1700;1800;1900;2000]  InternalRulePriority=Speed  RndMeth=Simplest
  Out1 : Outport
  wires:
  In1/1 -> LUT 1.11RR/1
  LUT 1.11RR/1 -> Out1/1

== system LUT_liver_pancreas_30/If Action Subsystem6/If Action Subsystem1/If Action Subsystem5/If Action Subsystem2 ==
  In1 : Inport
  Action Port : ActionPort  ActionPortLabel=else
  LUT 1.10RR : Lookup_n-D  NumberOfTableDimensions=1  BreakpointsForDimension1=[464.3473;512.4817;609.9172;707.7112;805.4156;903.0173;1000.538;1097.998;1195.413;1292.792;1390.144;1487.473;1584.785;1682.08;1779.36;1876.625;1973.872]  Table=[400;500;600;700;800;900;1000;1100;1200;1300;1400;1500;1600;1700;1800;1900;2000]  InternalRulePriority=Speed  RndMeth=Simplest
  Out1 : Outport
  wires:
  In1/1 -> LUT 1.10RR/1
  LUT 1.10RR/1 -> Out1/1

== system LUT_liver_pancreas_30/If Action Subsystem6/If Action Subsystem1/If Action Subsystem5/If Action Subsystem3 ==
  In1 : Inport
  Action Port : ActionPort  ActionPortLabel=elseif( u1 >= 1.125)
  LUT 1.13RR : Lookup_n-D  NumberOfTableDimensions=1  BreakpointsForDimension1=[463.8196;511.9183;609.1066;706.6261;804.0393;901.3389;998.5502;1095.695;1192.791;1289.849;1386.877;1483.882;1580.867;1677.836;1774.79;1871.729;1968.653]  Table=[400;500;600;700;800;900;1000;1100;1200;1300;1400;1500;1600;1700;1800;1900;2000]  InternalRulePriority=Speed  RndMeth=Simplest
  Out1 : Outport
  wires:
  In1/1 -> LUT 1.13RR/1
  LUT 1.13RR/1 -> Out1/1

== system LUT_liver_pancreas_30/If Action Subsystem6/If Action Subsystem1/If Action Subsystem5/If Action Subsystem4 ==
  In1 : Inport
  Action Port : ActionPort  ActionPortLabel=elseif( u1 >= 1.135)
  LUT 1.14RR : Lookup_n-D  NumberOfTableDimensions=1  BreakpointsForDimension1=[463.6493;511.7378;608.848;706.2804;803.601;900.8043;997.9167;1094.961;1191.955;1288.91;1385.835;1482.735;1579.616;1676.48;1773.329;1870.164;1966.983]  Table=[400;500;600;700;800;900;1000;1100;1200;1300;1400;1500;1600;1700;1800;1900;2000]  InternalRulePriority=Speed  RndMeth=Simplest
  Out1 : Outport
  wires:
  In1/1 -> LUT 1.14RR/1
  LUT 1.14RR/1 -> Out1/1

== system LUT_liver_pancreas_30/If Action Subsystem6/If Action Subsystem1/If Action Subsystem5/If Action Subsystem5 ==
  In1 : Inport
  Action Port : ActionPort  ActionPortLabel=elseif( u1 >= 1.155)
  LUT 1.16RR : Lookup_n-D  NumberOfTableDimensions=1  BreakpointsForDimension1=[463.3169;511.3872;608.3477;705.6123;802.7538;899.7706;996.6913;1093.541;1190.336;1287.092;1383.815;1480.513;1577.191;1673.851;1770.496;1867.128;1963.744]  Table=[400;500;600;700;800;900;1000;1100;1200;1300;1400;1500;1600;1700;1800;1900;2000]  InternalRulePriority=Speed  RndMeth=Simplest
  Out1 : Outport
  wires:
  In1/1 -> LUT 1.16RR/1
  LUT 1.16RR/1 -> Out1/1

== system LUT_liver_pancreas_30/If Action Subsystem6/If Action Subsystem1/If Action Subsystem5/If Action Subsystem6 ==
  In1 : Inport
  Action Port : ActionPort  ActionPortLabel=elseif( u1 >= 1.145)
  LUT 1.15RR : Lookup_n-D  NumberOfTableDimensions=1  BreakpointsForDimension1=[463.4817;511.5608;608.5951;705.9426;803.1726;900.2816;997.2972;1094.243;1191.137;1287.991;1384.814;1481.612;1578.391;1675.152;1771.898;1868.63;1965.347]  Table=[400;500;600;700;800;900;1000;1100;1200;1300;1400;1500;1600;1700;1800;1900;2000]  InternalRulePriority=Speed  RndMeth=Simplest
  Out1 : Outport
  wires:
  In1/1 -> LUT 1.15RR/1
  LUT 1.15RR/1 -> Out1/1

== system LUT_liver_pancreas_30/If Action Subsystem6/If Action Subsystem1/If Action Subsystem5/If Action Subsystem7 ==
  In1 : Inport
  Action Port : ActionPort  ActionPortLabel=elseif( u1 >= 1.165)
  LUT 1.17RR : Lookup_n-D  NumberOfTableDimensions=1  BreakpointsForDimension1=[463.1547;511.217;608.1057;705.2894;802.3443;899.2708;996.0987;1092.853;1189.553;1286.211;1382.837;1479.437;1576.016;1672.577;1769.123;1865.655;1962.173]  Table=[400;500;600;700;800;900;1000;1100;1200;1300;1400;1500;1600;1700;1800;1900;2000]  InternalRulePriority=Speed  RndMeth=Simplest
  Out1 : Outport
  wires:
  In1/1 -> LUT 1.17RR/1
  LUT 1.17RR/1 -> Out1/1

== system LUT_liver_pancreas_30/If Action Subsystem6/If Action Subsystem1/If Action Subsystem5/If Action Subsystem8 ==
  In1 : Inport
  Action Port : ActionPort  ActionPortLabel=elseif(u1 >= 1.175)
  LUT 1.18RR : Lookup_n-D  NumberOfTableDimensions=1  BreakpointsForDimension1=[462.9951;511.0501;607.869;704.9737;801.944;898.7822;995.5191;1092.181;1188.787;1285.349;1381.879;1478.383;1574.865;1671.329;1767.778;1864.213;1960.634]  Table=[400;500;600;700;800;900;1000;1100;1200;1300;1400;1500;1600;1700;1800;1900;2000]  InternalRulePriority=Speed  RndMeth=Simplest
  Out1 : Outport
  wires:
  In1/1 -> LUT 1.18RR/1
  LUT 1.18RR/1 -> Out1/1

== system LUT_liver_pancreas_30/If Action Subsystem6/If Action Subsystem1/If Action Subsystem5/If Action Subsystem9 ==
  In1 : Inport
  Action Port : ActionPort  ActionPortLabel=if(u1 >= 1.185)
  LUT 1.19RR : Lookup_n-D  NumberOfTableDimensions=1  BreakpointsForDimension1=[462.8381;510.8865;607.6374;704.665;801.5527;898.3043;994.9521;1091.523;1188.036;1284.506;1380.942;1477.35;1573.737;1670.106;1766.46;1862.799;1959.125]  Table=[400;500;600;700;800;900;1000;1100;1200;1300;1400;1500;1600;1700;1800;1900;2000]  InternalRulePriority=Speed  RndMeth=Simplest
  Out1 : Outport
  wires:
  In1/1 -> LUT 1.19RR/1
  LUT 1.19RR/1 -> Out1/1

== system LUT_liver_pancreas_30/If Action Subsystem6/If Action Subsystem1/If Action Subsystem6/If Action Subsystem1 ==
  In1 : Inport
  Action Port : ActionPort  ActionPortLabel=elseif( u1 >= 1.015)
  LUT 1.02RR : Lookup_n-D  NumberOfTableDimensions=1  BreakpointsForDimension1=[465.8818;514.1538;612.3582;710.9934;809.5822;908.0965;1006.549;1104.954;1203.323;1301.663;1399.981;1498.279;1596.56;1694.825;1793.073;1891.298;1989.483]  Table=[400;500;600;700;800;900;1000;1100;1200;1300;1400;1500;1600;1700;1800;1900;2000]  InternalRulePriority=Speed  RndMeth=Simplest
  Out1 : Outport
  wires:
  In1/1 -> LUT 1.02RR/1
  LUT 1.02RR/1 -> Out1/1

== system LUT_liver_pancreas_30/If Action Subsystem6/If Action Subsystem1/If Action Subsystem6/If Action Subsystem10 ==
  In1 : Inport
  Action Port : ActionPort  ActionPortLabel=elseif( u1 >= 1.005)
  LUT 1.01RR : Lookup_n-D  NumberOfTableDimensions=1  BreakpointsForDimension1=[466.0869;514.3811;612.6941;711.4469;810.1586;908.7992;1007.38;1105.916;1204.416;1302.888;1401.338;1499.769;1598.183;1696.58;1794.959;1893.314;1991.622]  Table=[400;500;600;700;800;900;1000;1100;1200;1300;1400;1500;1600;1700;1800;1900;2000]  InternalRulePriority=Speed  RndMeth=Simplest
  Out1 : Outport
  wires:
  In1/1 -> LUT 1.01RR/1
  LUT 1.01RR/1 -> Out1/1

== system LUT_liver_pancreas_30/If Action Subsystem6/If Action Subsystem1/If Action Subsystem6/If Action Subsystem2 ==
  In1 : Inport
  Action Port : ActionPort  ActionPortLabel=else
  LUT 1.00RR : Lookup_n-D  NumberOfTableDimensions=1  BreakpointsForDimension1=[466.295;514.6125;613.0372;711.9107;810.7482;909.518;1008.231;1106.899;1205.533;1304.14;1402.726;1501.292;1599.841;1698.374;1796.887;1895.373;1993.805]  Table=[400;500;600;700;800;900;1000;1100;1200;1300;1400;1500;1600;1700;1800;1900;2000]  InternalRulePriority=Speed  RndMeth=Simplest
  Out1 : Outport
  wires:
  In1/1 -> LUT 1.00RR/1
  LUT 1.00RR/1 -> Out1/1
